simulink model "pmsm_smo"  (R2025b)
settings: Solver=FixedStepDiscrete  StartTime=0.0  StopTime=15  FixedStep=50e-6  RelTol=1e-3  EnableMultiTasking=on
PostLoadFcn:
  | mchp_pmsm_foc_smo_dsPIC33_data;
InitFcn:
  | mchp_pmsm_foc_smo_dsPIC33_data;
values from neighbouring files (symbols this model uses):
  CalibId = 0    [mchp_pmsm_foc_smo_dsPIC33_data.m]
  CalibIq = 1.5    [mchp_pmsm_foc_smo_dsPIC33_data.m]
  CalibSpeed = 500    [mchp_pmsm_foc_smo_dsPIC33_data.m]
  CalibTime = 1/CalibFreq    (= 0.12)    [mchp_pmsm_foc_smo_dsPIC33_data.m]
  CalibVd = -0.7    [mchp_pmsm_foc_smo_dsPIC33_data.m]
  CalibVq = 2.69    [mchp_pmsm_foc_smo_dsPIC33_data.m]
  PI_Ki_id = (6.60e2)*Ts    (= 0.033)    [mchp_pmsm_foc_smo_dsPIC33_data.m]
  PI_Ki_iq = (6.60e2)*Ts    (= 0.033)    [mchp_pmsm_foc_smo_dsPIC33_data.m]
  PI_Ki_speed = (1.96e-6)    (= 1.96e-06)    [mchp_pmsm_foc_smo_dsPIC33_data.m]
  PI_Kp_id = 0.852    [mchp_pmsm_foc_smo_dsPIC33_data.m]
  PI_Kp_iq = 0.852    [mchp_pmsm_foc_smo_dsPIC33_data.m]
  PI_Kp_speed = 0.0062756    [mchp_pmsm_foc_smo_dsPIC33_data.m]
  PWM_frequency = 20e3    (= 20000)    [mchp_pmsm_foc_smo_dsPIC33_data.m]
  Ts = T_pwm    (= 5e-05)    [mchp_pmsm_foc_smo_dsPIC33_data.m]
  Ts_serialIn = 100e-3    (= 0.1)    [mchp_pmsm_foc_smo_dsPIC33_data.m]
  Ts_speed = 30*Ts    (= 0.0015)    [mchp_pmsm_foc_smo_dsPIC33_data.m]
undefined symbols (not defined in the file or in its folder): A0, A4, ADC, B0, C10, C11, C14, C15, C6, C7, C8, DiscIntNeverNeededParam, inverter, Max, MaxPer, ms, NumBits1, NumBits2, OpMode, P1, P17, P20, P39, P40, P41, P43, P44, P47, P48, Pin, pmsm, PWM1_Trg1, Resol, s, target, us
libraries: simulink x39, MCHP_Blockset x22, mcbeeMathTransformLib x7, mcbcontrolslib x7, slpidlib x5
(part 5 of 5)

== system pmsm_smo/Microcontroller/Application_Abstraction/SMO/Sliding Mode Observer/Subsystem4 ==
  θ : Inport
  w : Inport  Port=2
  Delay1 : Delay  DelayLength=1
  Discrete-Time Integrator4 : DiscreteIntegrator  IntegratorMethod=Integration: Backward Euler  SampleTime=-1  OutDataTypeStr=single  ICPrevOutput=DiscIntNeverNeededParam  ICPrevScaledInput=DiscIntNeverNeededParam
  Gain2 : Gain  Gain=0.3  OutDataTypeStr=single
  Gain3 : Gain  Gain=1/Ts  OutDataTypeStr=single
  Product1 : Product  OutDataTypeStr=single
  Sum2 : Sum  Inputs=|+-  OutDataTypeStr=single  AccumDataTypeStr=single
  Sum4 : Sum  Inputs=|+-  OutDataTypeStr=Inherit: Same as first input
  Unit Delay3 : UnitDelay  SampleTime=Ts  HasFrameUpgradeWarning=on
  Wrap_to_pi1 : Subsystem  VariantControl=VSS_STD
  Wrap_to_pi2 : Subsystem  VariantControl=VSS_STD
  ω_est : Outport  VectorParamsAs1DForOutWhenUnconnected=off
  θout : Outport  Port=2  VectorParamsAs1DForOutWhenUnconnected=off
  wires:
  Unit Delay3/1 -> Sum2/2
  θ/1 -> Wrap_to_pi1/1(θ), Sum2/1, Unit Delay3/1
  Sum4/1 -> Product1/2
  Product1/1 -> Discrete-Time Integrator4/1
  Delay1/1 -> Sum4/2
  Sum2/1 -> Wrap_to_pi2/1(θ)
  Discrete-Time Integrator4/1 -> ω_est/1, Delay1/1
  w/1 -> Gain2/1
  Gain2/1 -> Product1/1
  Gain3/1 -> Sum4/1
  Wrap_to_pi2/1(θ (-π,π)) -> Gain3/1
  Wrap_to_pi1/1(θ (-π,π)) -> θout/1

== system pmsm_smo/Microcontroller/Application_Abstraction/SMO/Sliding Mode Observer/atan1 ==
  note: Consistent with Microchip notation:
      |
      | x_α = cos(θ) * x_d - sin(θ) * x_q
      | x_β = sin(θ) * x_d + cos(θ) * x_q
      |
      | θ = atan2(sin(θ)/cos(θ)) = atan2(-x_α/x_β)
      |
      | provided x_d = 0, which is true in case of E_d
  α : Inport
  β : Inport  Port=2
  Bus Element In5 : Inport  Port=3  PortName=Calibdata  Element=Theta_Offset
  Bias2 : Bias  Bias=1.244  SaturateOnIntegerOverflow=off
  Gain3 : Gain  Gain=-1  OutDataTypeStr=Inherit: Same as input
  Subtract : Sum  Inputs=+-
  Trigonometric Function1 : Trigonometry  Operator=atan2  ApproximationMethod=Lookup  TableDataTypeStr=single
  θ : Outport  VectorParamsAs1DForOutWhenUnconnected=off
  wires:
  α/1 -> Gain3/1
  β/1 -> Trigonometric Function1/2
  Gain3/1 -> Trigonometric Function1/1
  Trigonometric Function1/1 -> Bias2/1
  Bias2/1 -> Subtract/1
  Subtract/1 -> θ/1
  Bus Element In5/1 -> Subtract/2

== system pmsm_smo/Microcontroller/Command_Signals/Command Signals/Codegen/Triggered Subsystem ==
  Trigger : TriggerPort  TriggerType=falling  VariantControl=Variant
  Delay : Delay  DelayLength=1  InitialCondition=0
  NOT : Logic  Operator=NOT  IconShape=distinctive  AllPortsSameDT=off  OutDataTypeStr=boolean
  RunCmd : Outport
  wires:
  NOT/1 -> RunCmd/1, Delay/1
  Delay/1 -> NOT/1

== system pmsm_smo/Microcontroller/Data Monitoring/SerialOutDrivers/codegen/SCI_Tx ==
  note: Fast Serial Data Monitoring (32-bit)
  Data_Log : Inport
  Constant : Constant  Value=target.frameSize -1  OutDataTypeStr=uint16
  Counter Limited : simulink/Sources/Counter Limited  uplimit=target.frameSize-1  tsamp=-1
  Data : Subsystem  TreatAsAtomicUnit=on
  Data Type Conversion : DataTypeConversion  OutDataTypeStr=uint16  RndMeth=Simplest  SaturateOnIntegerOverflow=off
  End : Subsystem  TreatAsAtomicUnit=on
  If : If  NumInputs=2  IfExpression=u1 == 0  ElseIfExpressions=u1 == u2
  Start : Subsystem  TreatAsAtomicUnit=on
  wires:
  If/3 -> Data/Action
  Counter Limited/1 -> Data Type Conversion/1
  If/2 -> End/Action
  If/1 -> Start/Action
  Data_Log/1 -> End/1(Data), Start/1(Data), Data/1(Data)
  Constant/1 -> If/2
  Data Type Conversion/1 -> If/1

== system pmsm_smo/Microcontroller/Application/Fast Task/Prepare/Init_Lock/Init ==
  Enable : EnablePort
  Constant10 : Constant  Value=[0 0 0]  OutDataTypeStr=dataType  SampleTime=Ts
  Vabc : Outport
  wires:
  Constant10/1 -> Vabc/1

== system pmsm_smo/Microcontroller/Application/Fast Task/Prepare/Init_Lock/Lock ==
  Enable : EnablePort
  Constant11 : Constant  Commented=on  Value=0.5  OutDataTypeStr=dataType  SampleTime=-1
  Constant2 : Constant  Value=[0.3 0.2 0.2]  OutDataTypeStr=dataType  SampleTime=Ts
  Constant3 : Constant  Commented=on  Value=0  OutDataTypeStr=Inherit: Inherit via back propagation  SampleTime=-1
  Constant4 : Constant  Commented=on  Value=0  OutDataTypeStr=Inherit: Inherit via back propagation  SampleTime=-1
  Constant5 : Constant  Commented=on  OutDataTypeStr=Inherit: Inherit via back propagation  SampleTime=-1
  Constant8 : Constant  Commented=on  Value=1.5  OutDataTypeStr=single  SampleTime=Ts
  Inverse Park Transform : mcbeeMathTransformLib/Park to Clarke Angle Transform  Commented=on  AxisAlignment=D-axis  UseWithEmbedded=on  PhaseInput=Two inputs  ThetaInput=Sine and Cosine electrical position  AngleInput=Per-unit  N_points=1024
  Mux2 : Mux  Commented=on  Inputs=3
  One_by_Two : Gain  Commented=on  Gain=1/(2*inverter.V_dc/sqrt(3))  RndMeth=Simplest  OutDataTypeStr=Inherit: Same as input
  Space Vector Generator : mcbcontrolslib/PWM Reference Generator  Commented=on  inSignal=Valphabeta  modType=SVM: space vector modulation
  Sum : Sum  Commented=on  Inputs=|++
  duty_cycles : Outport  VectorParamsAs1DForOutWhenUnconnected=off
  wires:
  Constant2/1 -> duty_cycles/1
  Space Vector Generator/2 -> Mux2/2
  Constant8/1 -> Inverse Park Transform/1
  Space Vector Generator/1 -> Mux2/1
  Constant5/1 -> Inverse Park Transform/4
  Space Vector Generator/3 -> Mux2/3
  Mux2/1 -> One_by_Two/1
  Inverse Park Transform/1 -> Space Vector Generator/1
  Inverse Park Transform/2 -> Space Vector Generator/2
  Constant4/1 -> Inverse Park Transform/3
  Constant11/1 -> Sum/2
  Constant3/1 -> Inverse Park Transform/2
  One_by_Two/1 -> Sum/1

== system pmsm_smo/Microcontroller/Application/Fast Task/Prepare/Init_Lock/Theta_Calib ==
  Enable : EnablePort
  Constant10 : Constant  Value=[0 0 0]  OutDataTypeStr=dataType  SampleTime=Ts
  Vabc : Outport
  wires:
  Constant10/1 -> Vabc/1

== system pmsm_smo/Microcontroller/Application/Fast Task/Prepare/Spin motor/Init ==
  Enable : EnablePort
  Constant1 : Constant  Value=0  OutDataTypeStr=boolean  SampleTime=Ts
  Constant10 : Constant  Value=0  OutDataTypeStr=boolean  SampleTime=Ts
  Constant2 : Constant  Value=0  OutDataTypeStr=dataType  SampleTime=Ts
  Theta_Check : Outport
  Speed_Check : Outport  Port=2
  Theta_offset : Outport  Port=3
  wires:
  Constant1/1 -> Theta_Check/1
  Constant10/1 -> Speed_Check/1
  Constant2/1 -> Theta_offset/1

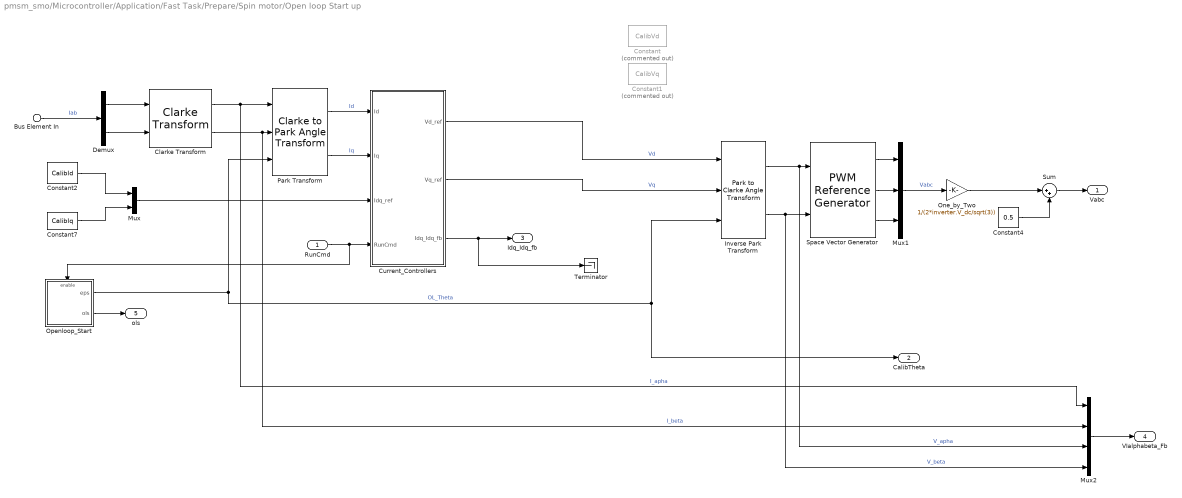
== system pmsm_smo/Microcontroller/Application/Fast Task/Prepare/Spin motor/Open loop Start up ==
  RunCmd : Inport
  Bus Element In : Inport  Port=2  PortName=HWInputs  Element=Iab
  Clarke Transform : mcbeeMathTransformLib/Clarke Transform  VariantControl=Variant2  PowerInvariant=off  UseWithEmbedded=on  PhaseInput=Two inputs
  Constant : Constant  Commented=on  Value=CalibVd  OutDataTypeStr=single  SampleTime=Ts
  Constant1 : Constant  Commented=on  Value=CalibVq  OutDataTypeStr=single  SampleTime=Ts
  Constant2 : Constant  Value=CalibId  OutDataTypeStr=single  SampleTime=Ts
  Constant4 : Constant  Value=0.5  OutDataTypeStr=dataType  SampleTime=-1
  Constant7 : Constant  Value=CalibIq  OutDataTypeStr=single  SampleTime=Ts
  Current_Controllers : Subsystem
  Demux : Demux  Outputs=2
  Inverse Park Transform : mcbeeMathTransformLib/Park to Clarke Angle Transform  AxisAlignment=D-axis  UseWithEmbedded=on  PhaseInput=Two inputs  ThetaInput=Electrical position  AngleInput=Radians  N_points=1024
  Mux : Mux  Inputs=2
  Mux1 : Mux  Inputs=3
  Mux2 : Mux
  One_by_Two : Gain  Gain=1/(2*inverter.V_dc/sqrt(3))  RndMeth=Simplest  OutDataTypeStr=Inherit: Same as input
  Openloop_Start : Subsystem
  Park Transform : mcbeeMathTransformLib/Clarke to Park Angle Transform  AxisAlignment=D-axis  UseWithEmbedded=on  PhaseInput=Two inputs  ThetaInput=Electrical position  AngleInput=Radians  N_points=1024
  Space Vector Generator : mcbcontrolslib/PWM Reference Generator  inSignal=Valphabeta  modType=SVM: space vector modulation
  Sum : Sum  Inputs=|++
  Terminator : Terminator
  Vabc : Outport  VectorParamsAs1DForOutWhenUnconnected=off
  CalibTheta : Outport  Port=2
  Idq_Idq_fb : Outport  Port=3  VectorParamsAs1DForOutWhenUnconnected=off
  VIalphabeta_Fb : Outport  Port=4
  ols : Outport  Port=5
  wires:
  Space Vector Generator/2 -> Mux1/2
  Space Vector Generator/3 -> Mux1/3
  Space Vector Generator/1 -> Mux1/1
  Constant4/1 -> Sum/2
  One_by_Two/1 -> Sum/1
  Mux1/1 -> One_by_Two/1  "Vabc"
  Sum/1 -> Vabc/1
  Inverse Park Transform/1 -> Mux2/3, Space Vector Generator/1  "V_apha"
  Inverse Park Transform/2 -> Space Vector Generator/2, Mux2/4  "V_beta"
  Demux/2 -> Clarke Transform/2
  RunCmd/1 -> Openloop_Start/Enable, Current_Controllers/4(RunCmd)
  Demux/1 -> Clarke Transform/1
  Park Transform/1 -> Current_Controllers/1(Id)  "Id"
  Mux/1 -> Current_Controllers/3(Idq_ref)
  Current_Controllers/3(Idq_Idq_fb) -> Terminator/1, Idq_Idq_fb/1
  Park Transform/2 -> Current_Controllers/2(Iq)  "Iq"
  Bus Element In/1 -> Demux/1  "Iab"
  Constant7/1 -> Mux/2
  Constant2/1 -> Mux/1
  Clarke Transform/1 -> Mux2/1, Park Transform/1  "I_apha"
  Clarke Transform/2 -> Mux2/2, Park Transform/2  "I_beta"
  Mux2/1 -> VIalphabeta_Fb/1
  Openloop_Start/1(eps) -> Inverse Park Transform/3, CalibTheta/1, Park Transform/3  "OL_Theta"
  Current_Controllers/1(Vd_ref) -> Inverse Park Transform/1  "Vd"
  Current_Controllers/2(Vq_ref) -> Inverse Park Transform/2  "Vq"
  Openloop_Start/2(ols) -> ols/1

== system pmsm_smo/Microcontroller/Application/Fast Task/Prepare/Spin motor/SpeedCheck ==
  In Bus Element : Inport  PortName=HWInputs  Element=SpeedRef
  In Bus Element1 : Inport  PortName=HWInputs  Element=Speed_SMO
  Enable : EnablePort
  Abs : Abs  SaturateOnIntegerOverflow=off
  Compare To Constant : simulink/Logic and Bit Operations/Compare To Constant  relop=<=  const=5  OutDataTypeStr=boolean
  Constant1 : Constant  Value=0  OutDataTypeStr=boolean  SampleTime=Ts
  Constant2 : Constant  Value=0  OutDataTypeStr=dataType  SampleTime=Ts
  Subtract : Sum  Inputs=+-
  Speed_Check : Outport
  Theta_Check : Outport  Port=2
  Theta_offset : Outport  Port=3
  wires:
  Subtract/1 -> Abs/1
  Abs/1 -> Compare To Constant/1
  Compare To Constant/1 -> Speed_Check/1
  In Bus Element/1 -> Subtract/1
  In Bus Element1/1 -> Subtract/2
  Constant1/1 -> Theta_Check/1
  Constant2/1 -> Theta_offset/1

== system pmsm_smo/Microcontroller/Application/Fast Task/Prepare/Spin motor/Theta_check ==
  In Bus Element3 : Inport  PortName=HWInputs  Element=Theta_SMO
  OL_Theta : Inport  Port=2
  Enable : EnablePort
  Abs1 : Abs  SaturateOnIntegerOverflow=off
  Compare To Constant1 : simulink/Logic and Bit Operations/Compare To Constant  relop=<=  const=0.08  OutDataTypeStr=boolean
  Constant10 : Constant  OutDataTypeStr=boolean  SampleTime=Ts
  Mux : Mux  Inputs=2
  Scope : Scope
      settings: ActiveDisplayYMinimum=-3.79216  ActiveDisplayYMaximum=3.16318  DataLoggingVariableName=ScopeData3
  Subtract1 : Sum  Inputs=+-
  Wrap_to_pi2 : Subsystem  VariantControl=VSS_STD
  Theta_offset : Outport
  Theta_Check : Outport  Port=2
  Speed_Check : Outport  Port=3
  wires:
  Subtract1/1 -> Wrap_to_pi2/1(θ)
  Abs1/1 -> Compare To Constant1/1
  OL_Theta/1 -> Subtract1/2, Mux/2  "OL_Theta"
  In Bus Element3/1 -> Mux/1, Subtract1/1
  Compare To Constant1/1 -> Theta_Check/1
  Wrap_to_pi2/1(θ (-π,π)) -> Abs1/1, Theta_offset/1
  Constant10/1 -> Speed_Check/1
  Mux/1 -> Scope/1

== system pmsm_smo/Microcontroller/Application/Fast Task/Run/Closedloop/Speed Control ==
  Speed_Meas : Inport
  RunCmd : Inport  Port=2
  Speed_Ref : Inport  Port=3
  Constant : Constant  Value=0  OutDataTypeStr=single
  Mux : Mux  Inputs=2
  PI_Controller_Speed : Subsystem
  IdqRef : Outport  VectorParamsAs1DForOutWhenUnconnected=off
  wires:
  Speed_Ref/1 -> PI_Controller_Speed/1(N_ref)  "Speed_Ref"
  Speed_Meas/1 -> PI_Controller_Speed/2(N_fb)  "Speed_fb"
  RunCmd/1 -> PI_Controller_Speed/3(RunCmd)
  Mux/1 -> IdqRef/1
  Constant/1 -> Mux/1
  PI_Controller_Speed/1(Iq_ref) -> Mux/2

== system pmsm_smo/Microcontroller/Application/Fast Task/Run/CurrentControl/Current_Controllers ==
  Id : Inport
  Iq : Inport  Port=2
  Idq_ref : Inport  Port=3
  RunCmd : Inport  Port=4
  DQ Limiter : mcbcontrolslib/DQ Limiter  satMethodInputType=Specify via dialog  satMethodSelected=D-Q equivalence  satLimitInputType=Specify via dialog  Vmax=inverter.V_dc/sqrt(3)
  Demux : Demux  Outputs=2
  Mux : Mux
  PI_Controller_Id : Subsystem
  PI_Controller_Iq : Subsystem
  Terminator : Terminator
  Vd_ref : Outport  VectorParamsAs1DForOutWhenUnconnected=off
  Vq_ref : Outport  Port=2  VectorParamsAs1DForOutWhenUnconnected=off
  Idq_Idq_fb : Outport  Port=3  VectorParamsAs1DForOutWhenUnconnected=off
  wires:
  RunCmd/1 -> PI_Controller_Iq/3(RunCmd), PI_Controller_Id/2(RunCmd)  "Enable"
  Mux/1 -> Idq_Idq_fb/1
  DQ Limiter/3 -> Terminator/1
  DQ Limiter/2 -> Vq_ref/1
  DQ Limiter/1 -> Vd_ref/1
  PI_Controller_Iq/1(V_ref) -> DQ Limiter/2
  PI_Controller_Id/1(V_ref) -> DQ Limiter/1
  Idq_ref/1 -> Demux/1
  Demux/2 -> PI_Controller_Iq/2(I_ref), Mux/3  "Iq_Ref"
  Demux/1 -> PI_Controller_Id/1(I_ref), Mux/1  "Id_Ref"
  Id/1 -> PI_Controller_Id/3(I_fb), Mux/2  "Id_fb"
  Iq/1 -> Mux/4, PI_Controller_Iq/1(I_fb)  "Iq_fb"

== system pmsm_smo/Microcontroller/Application_Abstraction/SMO/Sliding Mode Observer/Subsystem4/Wrap_to_pi1 ==
  note: Subtract pi
  note: What's left after
      | division by 2pi
      | again
  note: Add pi
  note: This block limits the output angle between +/- π.
  note: What's left after
      | division by 2pi
  θ : Inport
  Bias : Bias  Bias=pi  SaturateOnIntegerOverflow=off
  Bias1 : Bias  Bias=-pi  SaturateOnIntegerOverflow=off
  Math Function : Math  Operator=mod  SignedPower=on
  Math Function1 : Math  Operator=mod  SignedPower=on
  load torque1 : Constant  Value=2*pi  OutDataTypeStr=single  SampleTime=Ts
  θ (-π,π) : Outport  VectorParamsAs1DForOutWhenUnconnected=off
  wires:
  Bias1/1 -> θ (-π,π)/1
  Bias/1 -> Math Function/1
  load torque1/1 -> Math Function/2, Math Function1/2
  Math Function/1 -> Bias1/1
  θ/1 -> Math Function1/1
  Math Function1/1 -> Bias/1

== system pmsm_smo/Microcontroller/Application_Abstraction/SMO/Sliding Mode Observer/Subsystem4/Wrap_to_pi2 ==
  note: What's left after
      | division by 2pi
  note: This block limits the output angle between +/- π.
  note: Add pi
  note: What's left after
      | division by 2pi
      | again
  note: Subtract pi
  θ : Inport
  Bias : Bias  Bias=pi  SaturateOnIntegerOverflow=off
  Bias1 : Bias  Bias=-pi  SaturateOnIntegerOverflow=off
  Math Function : Math  Operator=mod  SignedPower=on
  Math Function1 : Math  Operator=mod  SignedPower=on
  load torque1 : Constant  Value=2*pi  OutDataTypeStr=single  SampleTime=Ts
  θ (-π,π) : Outport  VectorParamsAs1DForOutWhenUnconnected=off
  wires:
  Math Function1/1 -> Bias/1
  θ/1 -> Math Function1/1
  Math Function/1 -> Bias1/1
  load torque1/1 -> Math Function1/2, Math Function/2
  Bias/1 -> Math Function/1
  Bias1/1 -> θ (-π,π)/1

== system pmsm_smo/Microcontroller/Data Monitoring/SerialOutDrivers/codegen/SCI_Tx/Data ==
  Data : Inport
  Action Port : ActionPort  ActionPortLabel=else
  UART Tx : MCHP_Blockset/BUS UART/UART Tx  UART_REF=1  ORDERING=None  AllOrNothing=off  SampleTime=-1  MCHP_MASTERLINK=pmsm_smo/BOARD MCLV-48V-300W dsPIC33AK512MC510 MC DIM/Microchip Master  NSend_Input=off  UART_String=off  NSend_Output=off
      settings: SourceProductName=MPLAB Device Blocks for Simulink
  wires:
  Data/1 -> UART Tx/1

== system pmsm_smo/Microcontroller/Data Monitoring/SerialOutDrivers/codegen/SCI_Tx/End ==
  Data : Inport
  Action Port : ActionPort  ActionPortLabel=elseif(u1 == u2)
  Mux : Mux  Inputs=2
  Start : Constant  Value=hex2dec('45')  OutDataTypeStr=uint8
  UART Tx : MCHP_Blockset/BUS UART/UART Tx  UART_REF=1  ORDERING=None  AllOrNothing=off  SampleTime=-1  MCHP_MASTERLINK=pmsm_smo/BOARD MCLV-48V-300W dsPIC33AK512MC510 MC DIM/Microchip Master  NSend_Input=off  UART_String=off  NSend_Output=off
      settings: SourceProductName=MPLAB Device Blocks for Simulink
  wires:
  Mux/1 -> UART Tx/1
  Data/1 -> Mux/1
  Start/1 -> Mux/2

== system pmsm_smo/Microcontroller/Data Monitoring/SerialOutDrivers/codegen/SCI_Tx/Start ==
  Data : Inport
  Action Port : ActionPort  ActionPortLabel=if(u1 == 0)
  End : Constant  Value=hex2dec('53')  OutDataTypeStr=uint8
  Mux : Mux  Inputs=2
  UART Tx : MCHP_Blockset/BUS UART/UART Tx  UART_REF=1  ORDERING=None  AllOrNothing=off  SampleTime=-1  MCHP_MASTERLINK=pmsm_smo/BOARD MCLV-48V-300W dsPIC33AK512MC510 MC DIM/Microchip Master  NSend_Input=off  UART_String=off  NSend_Output=off
      settings: SourceProductName=MPLAB Device Blocks for Simulink
  wires:
  Mux/1 -> UART Tx/1
  Data/1 -> Mux/2
  End/1 -> Mux/1

== system pmsm_smo/Microcontroller/Application/Fast Task/Prepare/Spin motor/Open loop Start up/Current_Controllers ==
  Id : Inport
  Iq : Inport  Port=2
  Idq_ref : Inport  Port=3
  RunCmd : Inport  Port=4
  DQ Limiter : mcbcontrolslib/DQ Limiter  satMethodInputType=Specify via dialog  satMethodSelected=D-Q equivalence  satLimitInputType=Specify via dialog  Vmax=inverter.V_dc/sqrt(3)
  Demux : Demux  Outputs=2
  Mux : Mux
  PI_Controller_Id : Subsystem
  PI_Controller_Iq : Subsystem
  Terminator : Terminator
  Vd_ref : Outport  VectorParamsAs1DForOutWhenUnconnected=off
  Vq_ref : Outport  Port=2  VectorParamsAs1DForOutWhenUnconnected=off
  Idq_Idq_fb : Outport  Port=3  VectorParamsAs1DForOutWhenUnconnected=off
  wires:
  RunCmd/1 -> PI_Controller_Iq/3(RunCmd), PI_Controller_Id/2(RunCmd)  "Enable"
  Mux/1 -> Idq_Idq_fb/1
  DQ Limiter/3 -> Terminator/1
  DQ Limiter/2 -> Vq_ref/1
  DQ Limiter/1 -> Vd_ref/1
  PI_Controller_Iq/1(V_ref) -> DQ Limiter/2
  PI_Controller_Id/1(V_ref) -> DQ Limiter/1
  Idq_ref/1 -> Demux/1
  Demux/2 -> PI_Controller_Iq/2(I_ref), Mux/3  "Iq_Ref"
  Demux/1 -> PI_Controller_Id/1(I_ref), Mux/1  "Id_Ref"
  Id/1 -> PI_Controller_Id/3(I_fb), Mux/2  "Id_fb"
  Iq/1 -> Mux/4, PI_Controller_Iq/1(I_fb)  "Iq_fb"

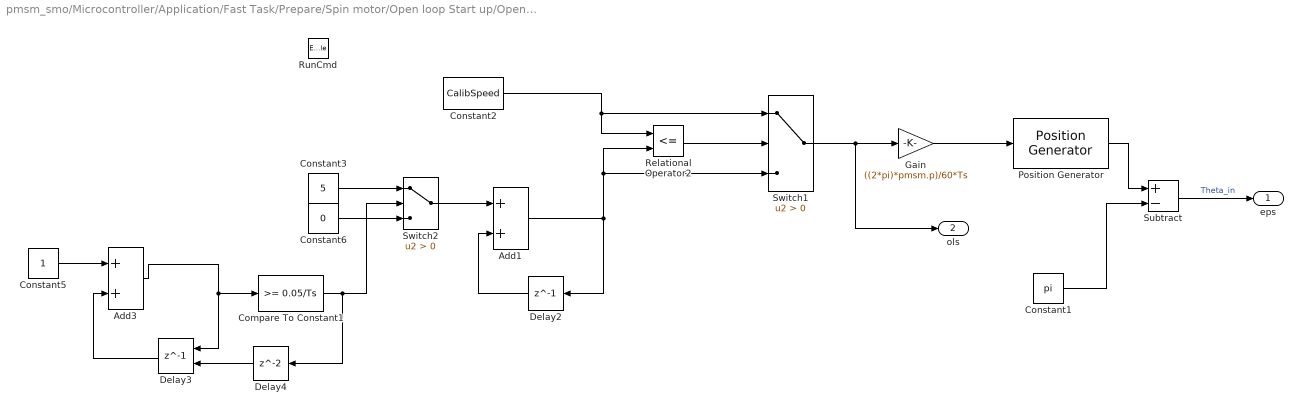
== system pmsm_smo/Microcontroller/Application/Fast Task/Prepare/Spin motor/Open loop Start up/Openloop_Start ==
  RunCmd : EnablePort  StatesWhenEnabling=reset
  Add1 : Sum  SaturateOnIntegerOverflow=on  OutDataTypeStr=Inherit: Same as first input
  Add3 : Sum  SaturateOnIntegerOverflow=on  OutDataTypeStr=Inherit: Same as first input
  Compare To Constant1 : simulink/Logic and Bit Operations/Compare To Constant  relop=>=  const=0.05/Ts  OutDataTypeStr=boolean
  Constant1 : Constant  Value=pi  OutDataTypeStr=single  SampleTime=Ts
  Constant2 : Constant  Value=CalibSpeed  OutDataTypeStr=single  SampleTime=Ts
  Constant3 : Constant  Value=5  OutDataTypeStr=single  SampleTime=Ts
  Constant5 : Constant  OutDataTypeStr=single  SampleTime=Ts
  Constant6 : Constant  Value=0  OutDataTypeStr=single  SampleTime=Ts
  Delay2 : Delay  DelayLength=1  InitialCondition=5
  Delay3 : Delay  DelayLength=1  ExternalReset=Rising
      settings: InputPortMap=u0,r5
  Delay4 : Delay  InitialCondition=5
  Gain : Gain  Gain=((2*pi)*pmsm.p)/60*Ts  OutDataTypeStr=single
  Position Generator : mcbcontrolslib/Position Generator  AngleOutput=Radians  InitialThetaSource=Specify via dialog  ExternalReset=none  Offset=0
  Relational Operator2 : RelationalOperator  Operator=<=  OutDataTypeStr=boolean  RndMeth=Simplest  InputSameDT=off
  Subtract : Sum  Inputs=+-
  Switch1 : Switch  Criteria=u2 > Threshold  SaturateOnIntegerOverflow=off  InputSameDT=off
  Switch2 : Switch  Criteria=u2 > Threshold  SaturateOnIntegerOverflow=off  InputSameDT=off
  eps : Outport
  ols : Outport  Port=2
  wires:
  Switch2/1 -> Add1/1
  Constant6/1 -> Switch2/3
  Compare To Constant1/1 -> Delay4/1, Switch2/2
  Gain/1 -> Position Generator/1
  Add3/1 -> Compare To Constant1/1, Delay3/1
  Delay2/1 -> Add1/2
  Constant5/1 -> Add3/1
  Constant2/1 -> Relational Operator2/1, Switch1/1
  Delay3/1 -> Add3/2
  Relational Operator2/1 -> Switch1/2
  Add1/1 -> Relational Operator2/2, Switch1/3, Delay2/1
  Constant3/1 -> Switch2/1
  Delay4/1 -> Delay3/2
  Position Generator/1 -> Subtract/1
  Constant1/1 -> Subtract/2
  Subtract/1 -> eps/1  "Theta_in"
  Switch1/1 -> ols/1, Gain/1

== system pmsm_smo/Microcontroller/Application/Fast Task/Prepare/Spin motor/Theta_check/Wrap_to_pi2 ==
  note: What's left after
      | division by 2pi
  note: This block limits the output angle between +/- π.
  note: Add pi
  note: What's left after
      | division by 2pi
      | again
  note: Subtract pi
  θ : Inport
  Bias : Bias  Bias=pi  SaturateOnIntegerOverflow=off
  Bias1 : Bias  Bias=-pi  SaturateOnIntegerOverflow=off
  Math Function : Math  Operator=mod  SignedPower=on
  Math Function1 : Math  Operator=mod  SignedPower=on
  load torque1 : Constant  Value=2*pi  OutDataTypeStr=single  SampleTime=Ts
  θ (-π,π) : Outport  VectorParamsAs1DForOutWhenUnconnected=off
  wires:
  Math Function1/1 -> Bias/1
  θ/1 -> Math Function1/1
  Math Function/1 -> Bias1/1
  load torque1/1 -> Math Function1/2, Math Function/2
  Bias/1 -> Math Function/1
  Bias1/1 -> θ (-π,π)/1

== system pmsm_smo/Microcontroller/Application/Fast Task/Run/Closedloop/Speed Control/PI_Controller_Speed ==
  N_ref : Inport
  N_fb : Inport  Port=2
  RunCmd : Inport  Port=3
  Discrete PI Controller with anti-windup & reset : slpidlib/PID Controller  Controller=PI  Form=Parallel  TimeDomain=Discrete-time  UseExternalTs=off  SampleTime=-1  IntegratorMethod=Forward Euler  FilterMethod=Forward Euler  ControllerParametersSource=external  P=1  I=1  UseKiTs=on  D=0  UseExternalDerivativeSource=off  N=100  UseFilter=on  TunerSelectOption=Transfer Function Based (PID Tuner App)  InitialConditionSource=external  InitialConditionForIntegrator=0  InitialConditionForFilter=0  DifferentiatorICPrevScaledInput=0  ExternalReset=level  TrackingMode=off  Kt=1  LimitOutput=on  SatLimitsSource=internal  UpperSaturationLimit=pmsm.I_rated  LowerSaturationLimit=-pmsm.I_rated  LinearizeAsGain=on  AntiWindupMode=clamping  Kb=1  LimitIntegrator=off  UpperIntegratorSaturationLimit=inf  LowerIntegratorSaturationLimit=-inf  RndMeth=Simplest  POutMin=[]  POutMax=[]  IOutMin=[]  IOutMax=[]  DOutMin=[]  DOutMax=[]  NOutMin=[]  NOutMax=[]  SumOutMin=[]  SumOutMax=[]  SaturationOutDataTypeStr=Inherit: Inherit via back propagation  SaturationOutMin=[]  SaturationOutMax=[]  PParamMin=[]  PParamMax=[]  IParamMin=[]  IParamMax=[]  DParamMin=[]  DParamMax=[]  NParamMin=[]  NParamMax=[]  KbParamMin=[]  KbParamMax=[]  KtParamMin=[]  KtParamMax=[]  KbOutMin=[]  KbOutMax=[]  KtOutMin=[]  KtOutMax=[]  IntegratorOutMin=[]  IntegratorOutMax=[]  FilterOutMin=[]  FilterOutMax=[]  SumI1OutMin=[]  SumI1OutMax=[]  SumI2OutMin=[]  SumI2OutMax=[]  SumI3OutMin=[]  SumI3OutMax=[]  SumI4OutMin=[]  SumI4OutMax=[]  SumDOutMin=[]  SumDOutMax=[]  DifferentiatorOutMin=[]  DifferentiatorOutMax=[]  FilterDiffOutCoefMin=[]  FilterDiffOutCoefMax=[]  ReciprocalOutMin=[]  ReciprocalOutMax=[]  SumDenOutMin=[]  SumDenOutMax=[]  SumNumOutMin=[]  SumNumOutMax=[]  DivideOutMin=[]  DivideOutMax=[]  UdiffTsProdOutMin=[]  UdiffTsProdOutMax=[]  NTsProdOutMin=[]  NTsProdOutMax=[]  UintegralTsProdOutMin=[]  UintegralTsProdOutMax=[]  UngainTsProdOutMin=[]  UngainTsProdOutMax=[]  ClampingZeroOutDataTypeStr=Inherit: Inherit via back propagation  ClampingZeroOutMin=[]  ClampingZeroOutMax=[]  FilterDenConstantOutDataTypeStr=Inherit: Inherit via back propagation  FilterDenConstantOutMin=[]  FilterDenConstantOutMax=[]  PCopyOutDataTypeStr=Inherit: Inherit via back propagation  PCopyOutMin=[]  PCopyOutMax=[]  NCopyOutDataTypeStr=Inherit: Inherit via back propagation  NCopyOutMin=[]  NCopyOutMax=[]  IntegratorContinuousStateAttributes=''  IntegratorStateMustResolveToSignalObject=off  IntegratorRTWStateStorageClass=Auto  FilterContinuousStateAttributes=''  FilterStateMustResolveToSignalObject=off  FilterRTWStateStorageClass=Auto  ParallelPVariant=ExternalParameters  IdealPVariant=Disabled  IVariant=ExternalParameters  DVariant=Disabled  IntegratorVariant=Discrete  SatVariant=Enabled  AWVariant=DiscClampingParallel  PCopyVariant=Disabled  TRVariant=Disabled  FdbkBlocksVariant=Forward  IdealPFdbkVariant=Disabled  SatFdbkVariant=Disabled  DerivativeFilterVariant=Disabled  NVariant=Disabled  NCopyVariant=Disabled_SignalSpec  FilterICVariant=Disabled  IntegratorICVariant=ExternalICs  ExternalResetVariant=ExternalReset  TRSumVariant=Passthrough  SumFdbkVariant=Disabled  SumVariant=Sum_PI  TsampFilterVariant=InternalTs  TsampNgainVariant=Passthrough  TsampIntegralVariant=Disabled_SignalSpec  ExternalSaturationOutDataTypeStr=Inherit: Same as second input  DerivativeSourceVariant=Disabled  PreIntVariant=InternalPreInt
  Ki2 : Constant  Value=0  OutDataTypeStr=single  SampleTime=-1
  Ki3 : Constant  Value=PI_Ki_speed*9.0658  OutDataTypeStr=single  SampleTime=-1
  Kp2 : Constant  Value=PI_Kp_speed*0.246667  OutDataTypeStr=single  SampleTime=Ts_speed
  Logical Operator : Logic  Operator=NOT  IconShape=distinctive  AllPortsSameDT=off  OutDataTypeStr=boolean
  Sum : Sum  Inputs=|+-  OutDataTypeStr=Inherit: Same as first input
  Zero_Cancellation : mcbcontrolslib/IIR Filter  VariantControl=Low Pass Filter  VariantSelect=Low-pass  FilterConstantInputType=Specify via dialog  Filter_constant=0.001*(Ts_speed/Ts)  InitialOutput=Specify via dialog  InitialOutputValue=0  ExternalReset=none  advancedSettings=off  Ts=50e-6  cutOff_freq=98.4464
  Iq_ref : Outport  VectorParamsAs1DForOutWhenUnconnected=off
  wires:
  Zero_Cancellation/1 -> Sum/1
  RunCmd/1 -> Logical Operator/1
  Ki2/1 -> Discrete PI Controller with anti-windup & reset/5
  Logical Operator/1 -> Discrete PI Controller with anti-windup & reset/4
  Sum/1 -> Discrete PI Controller with anti-windup & reset/1
  N_ref/1 -> Zero_Cancellation/1
  N_fb/1 -> Sum/2
  Kp2/1 -> Discrete PI Controller with anti-windup & reset/2
  Ki3/1 -> Discrete PI Controller with anti-windup & reset/3
  Discrete PI Controller with anti-windup & reset/1 -> Iq_ref/1

== system pmsm_smo/Microcontroller/Application/Fast Task/Run/CurrentControl/Current_Controllers/PI_Controller_Id ==
  I_ref : Inport
  RunCmd : Inport  Port=2
  I_fb : Inport  Port=3
  Discrete PI Controller with anti-windup & reset : slpidlib/PID Controller  Controller=PI  Form=Parallel  TimeDomain=Discrete-time  UseExternalTs=off  SampleTime=-1  IntegratorMethod=Forward Euler  FilterMethod=Forward Euler  ControllerParametersSource=external  P=1  I=1  UseKiTs=on  D=0  UseExternalDerivativeSource=off  N=100  UseFilter=on  TunerSelectOption=Transfer Function Based (PID Tuner App)  InitialConditionSource=external  InitialConditionForIntegrator=0  InitialConditionForFilter=0  DifferentiatorICPrevScaledInput=0  ExternalReset=level  TrackingMode=off  Kt=1  LimitOutput=on  SatLimitsSource=internal  UpperSaturationLimit=inverter.V_dc/sqrt(3)  LowerSaturationLimit=-inverter.V_dc/sqrt(3)  LinearizeAsGain=on  AntiWindupMode=clamping  Kb=1  LimitIntegrator=off  UpperIntegratorSaturationLimit=inf  LowerIntegratorSaturationLimit=-inf  RndMeth=Simplest  POutMin=[]  POutMax=[]  IOutMin=[]  IOutMax=[]  DOutMin=[]  DOutMax=[]  NOutMin=[]  NOutMax=[]  SumOutMin=[]  SumOutMax=[]  SaturationOutDataTypeStr=Inherit: Inherit via back propagation  SaturationOutMin=[]  SaturationOutMax=[]  PParamMin=[]  PParamMax=[]  IParamMin=[]  IParamMax=[]  DParamMin=[]  DParamMax=[]  NParamMin=[]  NParamMax=[]  KbParamMin=[]  KbParamMax=[]  KtParamMin=[]  KtParamMax=[]  KbOutMin=[]  KbOutMax=[]  KtOutMin=[]  KtOutMax=[]  IntegratorOutMin=[]  IntegratorOutMax=[]  FilterOutMin=[]  FilterOutMax=[]  SumI1OutMin=[]  SumI1OutMax=[]  SumI2OutMin=[]  SumI2OutMax=[]  SumI3OutMin=[]  SumI3OutMax=[]  SumI4OutMin=[]  SumI4OutMax=[]  SumDOutMin=[]  SumDOutMax=[]  DifferentiatorOutMin=[]  DifferentiatorOutMax=[]  FilterDiffOutCoefMin=[]  FilterDiffOutCoefMax=[]  ReciprocalOutMin=[]  ReciprocalOutMax=[]  SumDenOutMin=[]  SumDenOutMax=[]  SumNumOutMin=[]  SumNumOutMax=[]  DivideOutMin=[]  DivideOutMax=[]  UdiffTsProdOutMin=[]  UdiffTsProdOutMax=[]  NTsProdOutMin=[]  NTsProdOutMax=[]  UintegralTsProdOutMin=[]  UintegralTsProdOutMax=[]  UngainTsProdOutMin=[]  UngainTsProdOutMax=[]  ClampingZeroOutDataTypeStr=Inherit: Inherit via back propagation  ClampingZeroOutMin=[]  ClampingZeroOutMax=[]  FilterDenConstantOutDataTypeStr=Inherit: Inherit via back propagation  FilterDenConstantOutMin=[]  FilterDenConstantOutMax=[]  PCopyOutDataTypeStr=Inherit: Inherit via back propagation  PCopyOutMin=[]  PCopyOutMax=[]  NCopyOutDataTypeStr=Inherit: Inherit via back propagation  NCopyOutMin=[]  NCopyOutMax=[]  IntegratorContinuousStateAttributes=''  IntegratorStateMustResolveToSignalObject=off  IntegratorRTWStateStorageClass=Auto  FilterContinuousStateAttributes=''  FilterStateMustResolveToSignalObject=off  FilterRTWStateStorageClass=Auto  ParallelPVariant=ExternalParameters  IdealPVariant=Disabled  IVariant=ExternalParameters  DVariant=Disabled  IntegratorVariant=Discrete  SatVariant=Enabled  AWVariant=DiscClampingParallel  PCopyVariant=Disabled  TRVariant=Disabled  FdbkBlocksVariant=Forward  IdealPFdbkVariant=Disabled  SatFdbkVariant=Disabled  DerivativeFilterVariant=Disabled  NVariant=Disabled  NCopyVariant=Disabled_SignalSpec  FilterICVariant=Disabled  IntegratorICVariant=ExternalICs  ExternalResetVariant=ExternalReset  TRSumVariant=Passthrough  SumFdbkVariant=Disabled  SumVariant=Sum_PI  TsampFilterVariant=InternalTs  TsampNgainVariant=Passthrough  TsampIntegralVariant=Disabled_SignalSpec  ExternalSaturationOutDataTypeStr=Inherit: Same as second input  DerivativeSourceVariant=Disabled  PreIntVariant=InternalPreInt
  Ki : Constant  Value=PI_Ki_id  OutDataTypeStr=single  SampleTime=Ts
  Ki1 : Constant  Value=0  OutDataTypeStr=single  SampleTime=-1
  Kp : Constant  Value=PI_Kp_id  OutDataTypeStr=single  SampleTime=Ts
  Logical Operator : Logic  Operator=NOT  IconShape=distinctive  AllPortsSameDT=off  OutDataTypeStr=boolean
  Sum : Sum  Inputs=|+-  OutDataTypeStr=Inherit: Same as first input
  V_ref : Outport  VectorParamsAs1DForOutWhenUnconnected=off
  wires:
  Ki1/1 -> Discrete PI Controller with anti-windup & reset/5
  Logical Operator/1 -> Discrete PI Controller with anti-windup & reset/4
  Ki/1 -> Discrete PI Controller with anti-windup & reset/3
  Kp/1 -> Discrete PI Controller with anti-windup & reset/2
  Sum/1 -> Discrete PI Controller with anti-windup & reset/1
  Discrete PI Controller with anti-windup & reset/1 -> V_ref/1
  RunCmd/1 -> Logical Operator/1
  I_fb/1 -> Sum/2
  I_ref/1 -> Sum/1

== system pmsm_smo/Microcontroller/Application/Fast Task/Run/CurrentControl/Current_Controllers/PI_Controller_Iq ==
  I_fb : Inport
  I_ref : Inport  Port=2
  RunCmd : Inport  Port=3
  Discrete PI Controller with anti-windup & reset : slpidlib/PID Controller  Controller=PI  Form=Parallel  TimeDomain=Discrete-time  UseExternalTs=off  SampleTime=-1  IntegratorMethod=Forward Euler  FilterMethod=Forward Euler  ControllerParametersSource=external  P=1  I=1  UseKiTs=on  D=0  UseExternalDerivativeSource=off  N=100  UseFilter=on  TunerSelectOption=Transfer Function Based (PID Tuner App)  InitialConditionSource=external  InitialConditionForIntegrator=0  InitialConditionForFilter=0  DifferentiatorICPrevScaledInput=0  ExternalReset=level  TrackingMode=off  Kt=1  LimitOutput=on  SatLimitsSource=internal  UpperSaturationLimit=inverter.V_dc/sqrt(3)  LowerSaturationLimit=-inverter.V_dc/sqrt(3)  LinearizeAsGain=on  AntiWindupMode=clamping  Kb=1  LimitIntegrator=off  UpperIntegratorSaturationLimit=inf  LowerIntegratorSaturationLimit=-inf  RndMeth=Simplest  POutMin=[]  POutMax=[]  IOutMin=[]  IOutMax=[]  DOutMin=[]  DOutMax=[]  NOutMin=[]  NOutMax=[]  SumOutMin=[]  SumOutMax=[]  SaturationOutDataTypeStr=Inherit: Inherit via back propagation  SaturationOutMin=[]  SaturationOutMax=[]  PParamMin=[]  PParamMax=[]  IParamMin=[]  IParamMax=[]  DParamMin=[]  DParamMax=[]  NParamMin=[]  NParamMax=[]  KbParamMin=[]  KbParamMax=[]  KtParamMin=[]  KtParamMax=[]  KbOutMin=[]  KbOutMax=[]  KtOutMin=[]  KtOutMax=[]  IntegratorOutMin=[]  IntegratorOutMax=[]  FilterOutMin=[]  FilterOutMax=[]  SumI1OutMin=[]  SumI1OutMax=[]  SumI2OutMin=[]  SumI2OutMax=[]  SumI3OutMin=[]  SumI3OutMax=[]  SumI4OutMin=[]  SumI4OutMax=[]  SumDOutMin=[]  SumDOutMax=[]  DifferentiatorOutMin=[]  DifferentiatorOutMax=[]  FilterDiffOutCoefMin=[]  FilterDiffOutCoefMax=[]  ReciprocalOutMin=[]  ReciprocalOutMax=[]  SumDenOutMin=[]  SumDenOutMax=[]  SumNumOutMin=[]  SumNumOutMax=[]  DivideOutMin=[]  DivideOutMax=[]  UdiffTsProdOutMin=[]  UdiffTsProdOutMax=[]  NTsProdOutMin=[]  NTsProdOutMax=[]  UintegralTsProdOutMin=[]  UintegralTsProdOutMax=[]  UngainTsProdOutMin=[]  UngainTsProdOutMax=[]  ClampingZeroOutDataTypeStr=Inherit: Inherit via back propagation  ClampingZeroOutMin=[]  ClampingZeroOutMax=[]  FilterDenConstantOutDataTypeStr=Inherit: Inherit via back propagation  FilterDenConstantOutMin=[]  FilterDenConstantOutMax=[]  PCopyOutDataTypeStr=Inherit: Inherit via back propagation  PCopyOutMin=[]  PCopyOutMax=[]  NCopyOutDataTypeStr=Inherit: Inherit via back propagation  NCopyOutMin=[]  NCopyOutMax=[]  IntegratorContinuousStateAttributes=''  IntegratorStateMustResolveToSignalObject=off  IntegratorRTWStateStorageClass=Auto  FilterContinuousStateAttributes=''  FilterStateMustResolveToSignalObject=off  FilterRTWStateStorageClass=Auto  ParallelPVariant=ExternalParameters  IdealPVariant=Disabled  IVariant=ExternalParameters  DVariant=Disabled  IntegratorVariant=Discrete  SatVariant=Enabled  AWVariant=DiscClampingParallel  PCopyVariant=Disabled  TRVariant=Disabled  FdbkBlocksVariant=Forward  IdealPFdbkVariant=Disabled  SatFdbkVariant=Disabled  DerivativeFilterVariant=Disabled  NVariant=Disabled  NCopyVariant=Disabled_SignalSpec  FilterICVariant=Disabled  IntegratorICVariant=ExternalICs  ExternalResetVariant=ExternalReset  TRSumVariant=Passthrough  SumFdbkVariant=Disabled  SumVariant=Sum_PI  TsampFilterVariant=InternalTs  TsampNgainVariant=Passthrough  TsampIntegralVariant=Disabled_SignalSpec  ExternalSaturationOutDataTypeStr=Inherit: Same as second input  DerivativeSourceVariant=Disabled  PreIntVariant=InternalPreInt
  Ki : Constant  Value=PI_Ki_iq  OutDataTypeStr=single  SampleTime=Ts
  Kp : Constant  Value=PI_Kp_iq  OutDataTypeStr=single  SampleTime=Ts
  Kp1 : Constant  Value=0  OutDataTypeStr=single  SampleTime=-1
  Logical Operator : Logic  Operator=NOT  IconShape=distinctive  AllPortsSameDT=off  OutDataTypeStr=boolean
  Sum : Sum  Inputs=|+-  OutDataTypeStr=Inherit: Same as first input
  V_ref : Outport  VectorParamsAs1DForOutWhenUnconnected=off
  wires:
  RunCmd/1 -> Logical Operator/1
  Kp1/1 -> Discrete PI Controller with anti-windup & reset/5
  Logical Operator/1 -> Discrete PI Controller with anti-windup & reset/4
  Ki/1 -> Discrete PI Controller with anti-windup & reset/3
  Sum/1 -> Discrete PI Controller with anti-windup & reset/1
  Kp/1 -> Discrete PI Controller with anti-windup & reset/2
  I_ref/1 -> Sum/1
  I_fb/1 -> Sum/2
  Discrete PI Controller with anti-windup & reset/1 -> V_ref/1

== system pmsm_smo/Microcontroller/Application/Fast Task/Prepare/Spin motor/Open loop Start up/Current_Controllers/PI_Controller_Id ==
  I_ref : Inport
  RunCmd : Inport  Port=2
  I_fb : Inport  Port=3
  Discrete PI Controller with anti-windup & reset : slpidlib/PID Controller  Controller=PI  Form=Parallel  TimeDomain=Discrete-time  UseExternalTs=off  SampleTime=-1  IntegratorMethod=Forward Euler  FilterMethod=Forward Euler  ControllerParametersSource=external  P=1  I=1  UseKiTs=on  D=0  UseExternalDerivativeSource=off  N=100  UseFilter=on  TunerSelectOption=Transfer Function Based (PID Tuner App)  InitialConditionSource=external  InitialConditionForIntegrator=0  InitialConditionForFilter=0  DifferentiatorICPrevScaledInput=0  ExternalReset=level  TrackingMode=off  Kt=1  LimitOutput=on  SatLimitsSource=internal  UpperSaturationLimit=inverter.V_dc/sqrt(3)  LowerSaturationLimit=-inverter.V_dc/sqrt(3)  LinearizeAsGain=on  AntiWindupMode=clamping  Kb=1  LimitIntegrator=off  UpperIntegratorSaturationLimit=inf  LowerIntegratorSaturationLimit=-inf  RndMeth=Simplest  POutMin=[]  POutMax=[]  IOutMin=[]  IOutMax=[]  DOutMin=[]  DOutMax=[]  NOutMin=[]  NOutMax=[]  SumOutMin=[]  SumOutMax=[]  SaturationOutDataTypeStr=Inherit: Inherit via back propagation  SaturationOutMin=[]  SaturationOutMax=[]  PParamMin=[]  PParamMax=[]  IParamMin=[]  IParamMax=[]  DParamMin=[]  DParamMax=[]  NParamMin=[]  NParamMax=[]  KbParamMin=[]  KbParamMax=[]  KtParamMin=[]  KtParamMax=[]  KbOutMin=[]  KbOutMax=[]  KtOutMin=[]  KtOutMax=[]  IntegratorOutMin=[]  IntegratorOutMax=[]  FilterOutMin=[]  FilterOutMax=[]  SumI1OutMin=[]  SumI1OutMax=[]  SumI2OutMin=[]  SumI2OutMax=[]  SumI3OutMin=[]  SumI3OutMax=[]  SumI4OutMin=[]  SumI4OutMax=[]  SumDOutMin=[]  SumDOutMax=[]  DifferentiatorOutMin=[]  DifferentiatorOutMax=[]  FilterDiffOutCoefMin=[]  FilterDiffOutCoefMax=[]  ReciprocalOutMin=[]  ReciprocalOutMax=[]  SumDenOutMin=[]  SumDenOutMax=[]  SumNumOutMin=[]  SumNumOutMax=[]  DivideOutMin=[]  DivideOutMax=[]  UdiffTsProdOutMin=[]  UdiffTsProdOutMax=[]  NTsProdOutMin=[]  NTsProdOutMax=[]  UintegralTsProdOutMin=[]  UintegralTsProdOutMax=[]  UngainTsProdOutMin=[]  UngainTsProdOutMax=[]  ClampingZeroOutDataTypeStr=Inherit: Inherit via back propagation  ClampingZeroOutMin=[]  ClampingZeroOutMax=[]  FilterDenConstantOutDataTypeStr=Inherit: Inherit via back propagation  FilterDenConstantOutMin=[]  FilterDenConstantOutMax=[]  PCopyOutDataTypeStr=Inherit: Inherit via back propagation  PCopyOutMin=[]  PCopyOutMax=[]  NCopyOutDataTypeStr=Inherit: Inherit via back propagation  NCopyOutMin=[]  NCopyOutMax=[]  IntegratorContinuousStateAttributes=''  IntegratorStateMustResolveToSignalObject=off  IntegratorRTWStateStorageClass=Auto  FilterContinuousStateAttributes=''  FilterStateMustResolveToSignalObject=off  FilterRTWStateStorageClass=Auto  ParallelPVariant=ExternalParameters  IdealPVariant=Disabled  IVariant=ExternalParameters  DVariant=Disabled  IntegratorVariant=Discrete  SatVariant=Enabled  AWVariant=DiscClampingParallel  PCopyVariant=Disabled  TRVariant=Disabled  FdbkBlocksVariant=Forward  IdealPFdbkVariant=Disabled  SatFdbkVariant=Disabled  DerivativeFilterVariant=Disabled  NVariant=Disabled  NCopyVariant=Disabled_SignalSpec  FilterICVariant=Disabled  IntegratorICVariant=ExternalICs  ExternalResetVariant=ExternalReset  TRSumVariant=Passthrough  SumFdbkVariant=Disabled  SumVariant=Sum_PI  TsampFilterVariant=InternalTs  TsampNgainVariant=Passthrough  TsampIntegralVariant=Disabled_SignalSpec  ExternalSaturationOutDataTypeStr=Inherit: Same as second input  DerivativeSourceVariant=Disabled  PreIntVariant=InternalPreInt
  Ki : Constant  Value=PI_Ki_id  OutDataTypeStr=single  SampleTime=Ts
  Ki1 : Constant  Value=0  OutDataTypeStr=single  SampleTime=-1
  Kp : Constant  Value=PI_Kp_id  OutDataTypeStr=single  SampleTime=Ts
  Logical Operator : Logic  Operator=NOT  IconShape=distinctive  AllPortsSameDT=off  OutDataTypeStr=boolean
  Sum : Sum  Inputs=|+-  OutDataTypeStr=Inherit: Same as first input
  V_ref : Outport  VectorParamsAs1DForOutWhenUnconnected=off
  wires:
  Ki1/1 -> Discrete PI Controller with anti-windup & reset/5
  Logical Operator/1 -> Discrete PI Controller with anti-windup & reset/4
  Ki/1 -> Discrete PI Controller with anti-windup & reset/3
  Kp/1 -> Discrete PI Controller with anti-windup & reset/2
  Sum/1 -> Discrete PI Controller with anti-windup & reset/1
  Discrete PI Controller with anti-windup & reset/1 -> V_ref/1
  RunCmd/1 -> Logical Operator/1
  I_fb/1 -> Sum/2
  I_ref/1 -> Sum/1

== system pmsm_smo/Microcontroller/Application/Fast Task/Prepare/Spin motor/Open loop Start up/Current_Controllers/PI_Controller_Iq ==
  I_fb : Inport
  I_ref : Inport  Port=2
  RunCmd : Inport  Port=3
  Discrete PI Controller with anti-windup & reset : slpidlib/PID Controller  Controller=PI  Form=Parallel  TimeDomain=Discrete-time  UseExternalTs=off  SampleTime=-1  IntegratorMethod=Forward Euler  FilterMethod=Forward Euler  ControllerParametersSource=external  P=1  I=1  UseKiTs=on  D=0  UseExternalDerivativeSource=off  N=100  UseFilter=on  TunerSelectOption=Transfer Function Based (PID Tuner App)  InitialConditionSource=external  InitialConditionForIntegrator=0  InitialConditionForFilter=0  DifferentiatorICPrevScaledInput=0  ExternalReset=level  TrackingMode=off  Kt=1  LimitOutput=on  SatLimitsSource=internal  UpperSaturationLimit=inverter.V_dc/sqrt(3)  LowerSaturationLimit=-inverter.V_dc/sqrt(3)  LinearizeAsGain=on  AntiWindupMode=clamping  Kb=1  LimitIntegrator=off  UpperIntegratorSaturationLimit=inf  LowerIntegratorSaturationLimit=-inf  RndMeth=Simplest  POutMin=[]  POutMax=[]  IOutMin=[]  IOutMax=[]  DOutMin=[]  DOutMax=[]  NOutMin=[]  NOutMax=[]  SumOutMin=[]  SumOutMax=[]  SaturationOutDataTypeStr=Inherit: Inherit via back propagation  SaturationOutMin=[]  SaturationOutMax=[]  PParamMin=[]  PParamMax=[]  IParamMin=[]  IParamMax=[]  DParamMin=[]  DParamMax=[]  NParamMin=[]  NParamMax=[]  KbParamMin=[]  KbParamMax=[]  KtParamMin=[]  KtParamMax=[]  KbOutMin=[]  KbOutMax=[]  KtOutMin=[]  KtOutMax=[]  IntegratorOutMin=[]  IntegratorOutMax=[]  FilterOutMin=[]  FilterOutMax=[]  SumI1OutMin=[]  SumI1OutMax=[]  SumI2OutMin=[]  SumI2OutMax=[]  SumI3OutMin=[]  SumI3OutMax=[]  SumI4OutMin=[]  SumI4OutMax=[]  SumDOutMin=[]  SumDOutMax=[]  DifferentiatorOutMin=[]  DifferentiatorOutMax=[]  FilterDiffOutCoefMin=[]  FilterDiffOutCoefMax=[]  ReciprocalOutMin=[]  ReciprocalOutMax=[]  SumDenOutMin=[]  SumDenOutMax=[]  SumNumOutMin=[]  SumNumOutMax=[]  DivideOutMin=[]  DivideOutMax=[]  UdiffTsProdOutMin=[]  UdiffTsProdOutMax=[]  NTsProdOutMin=[]  NTsProdOutMax=[]  UintegralTsProdOutMin=[]  UintegralTsProdOutMax=[]  UngainTsProdOutMin=[]  UngainTsProdOutMax=[]  ClampingZeroOutDataTypeStr=Inherit: Inherit via back propagation  ClampingZeroOutMin=[]  ClampingZeroOutMax=[]  FilterDenConstantOutDataTypeStr=Inherit: Inherit via back propagation  FilterDenConstantOutMin=[]  FilterDenConstantOutMax=[]  PCopyOutDataTypeStr=Inherit: Inherit via back propagation  PCopyOutMin=[]  PCopyOutMax=[]  NCopyOutDataTypeStr=Inherit: Inherit via back propagation  NCopyOutMin=[]  NCopyOutMax=[]  IntegratorContinuousStateAttributes=''  IntegratorStateMustResolveToSignalObject=off  IntegratorRTWStateStorageClass=Auto  FilterContinuousStateAttributes=''  FilterStateMustResolveToSignalObject=off  FilterRTWStateStorageClass=Auto  ParallelPVariant=ExternalParameters  IdealPVariant=Disabled  IVariant=ExternalParameters  DVariant=Disabled  IntegratorVariant=Discrete  SatVariant=Enabled  AWVariant=DiscClampingParallel  PCopyVariant=Disabled  TRVariant=Disabled  FdbkBlocksVariant=Forward  IdealPFdbkVariant=Disabled  SatFdbkVariant=Disabled  DerivativeFilterVariant=Disabled  NVariant=Disabled  NCopyVariant=Disabled_SignalSpec  FilterICVariant=Disabled  IntegratorICVariant=ExternalICs  ExternalResetVariant=ExternalReset  TRSumVariant=Passthrough  SumFdbkVariant=Disabled  SumVariant=Sum_PI  TsampFilterVariant=InternalTs  TsampNgainVariant=Passthrough  TsampIntegralVariant=Disabled_SignalSpec  ExternalSaturationOutDataTypeStr=Inherit: Same as second input  DerivativeSourceVariant=Disabled  PreIntVariant=InternalPreInt
  Ki : Constant  Value=PI_Ki_iq  OutDataTypeStr=single  SampleTime=Ts
  Kp : Constant  Value=PI_Kp_iq  OutDataTypeStr=single  SampleTime=Ts
  Kp1 : Constant  Value=0  OutDataTypeStr=single  SampleTime=-1
  Logical Operator : Logic  Operator=NOT  IconShape=distinctive  AllPortsSameDT=off  OutDataTypeStr=boolean
  Sum : Sum  Inputs=|+-  OutDataTypeStr=Inherit: Same as first input
  V_ref : Outport  VectorParamsAs1DForOutWhenUnconnected=off
  wires:
  RunCmd/1 -> Logical Operator/1
  Kp1/1 -> Discrete PI Controller with anti-windup & reset/5
  Logical Operator/1 -> Discrete PI Controller with anti-windup & reset/4
  Ki/1 -> Discrete PI Controller with anti-windup & reset/3
  Sum/1 -> Discrete PI Controller with anti-windup & reset/1
  Kp/1 -> Discrete PI Controller with anti-windup & reset/2
  I_ref/1 -> Sum/1
  I_fb/1 -> Sum/2
  Discrete PI Controller with anti-windup & reset/1 -> V_ref/1

== stateflow chart pmsm_smo/Microcontroller/Application/Fast Task/Prepare/Init_Lock/Rotor Locking ==
  state Lock
    state Init
      entry:
      Lock = uint16(0);
    state ipsOffsetCalib
      entry:
      Lock = uint16(1);
    state Done
      during:
      Lock = uint16(0);
      Init_LockStatus = true;
    (default) -> Lock.Init
    Lock.Init -> ipsOffsetCalib
    ipsOffsetCalib -> Done : after(1,sec)
  state Init
    entry:
    Lock = uint16(0);
    Init_LockStatus = false;
  (default) -> Init
  Init -> Lock : [RunCmd == true]
  Lock -> Init : [RunCmd == false]
  data: Lock output; Init_LockStatus output; RunCmd input

== stateflow chart pmsm_smo/Microcontroller/Application/Fast Task/Calibration State ==
  state Calibration
    state Init_Lock
      entry:
      CalibMode = uint16(1);
      CalibStatus =false
    state ipsOffsetCalib
      entry:
      CalibMode = uint16(2);
      CalibStatus = false
    state Done
      entry:
      CalibMode = uint16(2);
      CalibStatus = true;
    (default) -> Init_Lock
    Init_Lock -> ipsOffsetCalib : [Init_LockStatus == true]
    ipsOffsetCalib -> Done : [after(CalibTime,sec)&&(Closedloop_Status==true)]
  state Init
    entry:
    CalibMode = uint16(1);
    CalibStatus = false;
  (default) -> Init
  Init -> Calibration : [RunCmd == true]
  Calibration -> Init : [RunCmd == false]
  data: RunCmd input; CalibTime input; CalibMode output; CalibStatus output; Init_LockStatus input; Closedloop_Status input

== stateflow chart pmsm_smo/Microcontroller/Application/Fast Task/Error Checking ==
  state Calibration
    state Start
      entry:
      Openloop_Mode = uint16(1);
      ClosedLoop_Status = false
    state ThetaOffsetCalib
      entry:
      Openloop_Mode = uint16(2);
      ClosedLoop_Status = false
    state Done
      during:
      Openloop_Mode = uint16(0);
      ClosedLoop_Status = true;
    (default) -> Start
    Start -> ThetaOffsetCalib : [Speed_Status == true]
    ThetaOffsetCalib -> Done : [(Theta_Status == true)]
  state Init
    entry:
    Openloop_Mode = uint16(1);
    ClosedLoop_Status = false;
  (default) -> Init
  Init -> Calibration : [RunCmd == true]
  Calibration -> Init : [RunCmd == false]
  data: RunCmd input; Speed_Status input; Theta_Status input; Openloop_Mode output; ClosedLoop_Status output

== stateflow chart pmsm_smo/Microcontroller/Application/System Mode Control/System Control ==
  state CurrOffsetCalib
    entry:
    Mode = OpMode.Inactive;
    CurrOffsetMeas = false;
  state Init
    entry:
    Mode = OpMode.Inactive;
    CurrOffsetMeas = true;
  state Prepare
    entry:
    Mode = OpMode.Prepare;
  state Run
    entry:
    Mode = OpMode.Run;
  (default) -> Init
  Prepare -> Run [order 1] : [(RunCmd == true) && (MotorReady == true)]
  CurrOffsetCalib -> Prepare : [RunCmd == true]
  Init -> CurrOffsetCalib : [after(0.5,sec)]
  Run -> Prepare : [RunCmd == false]
  Prepare -> CurrOffsetCalib [order 2] : [RunCmd == false]
  data: RunCmd input; Mode output Enum: OpMode =OpMode.Inactive; MotorReady input; CurrOffsetMeas output
